simulink model "lab2_2"  (R2025b)
settings: Solver=FixedStepAuto  StartTime=0.0  StopTime=50.0  FixedStep=2^-7  RelTol=1e-3
settings Model: Creator=mizula  LastModifiedBy=mizula

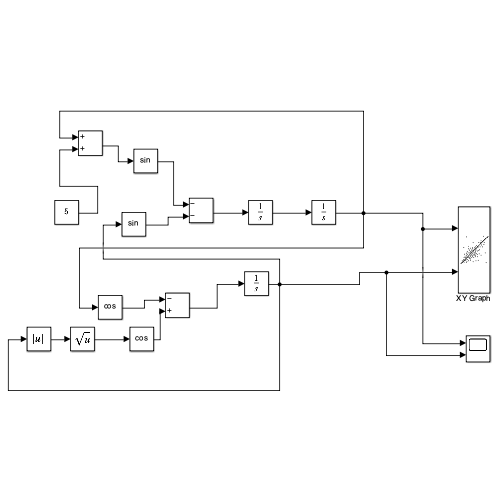
[thumbnail: Simulink's stored preview of the top-level diagram]
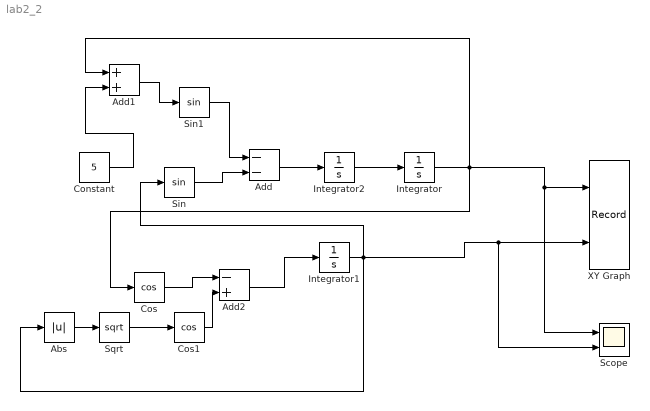
== system lab2_2 ==
  Abs : Abs  SaturateOnIntegerOverflow=off
  Add : Sum  Inputs=--
  Add1 : Sum
  Add2 : Sum  Inputs=-+
  Constant : Constant  Value=5
  Cos : Trigonometry  Operator=cos
  Cos1 : Trigonometry  Operator=cos
  Integrator : Integrator  InitialCondition=1
  Integrator1 : Integrator  InitialCondition=2
  Integrator2 : Integrator  InitialCondition=5
  Scope : Scope  NumInputPorts=2
      settings: ActiveDisplayYMinimum=-181.93688908773905  ActiveDisplayYMaximum=71.777306513933709
  Sin : Trigonometry
  Sin1 : Trigonometry
  Sqrt : Sqrt
  XY Graph : Record  NumPorts=2.0  FileSettingsInternal="{\"entries\":[{\"content\":{\"excelSettings\":{\"content\":{},\"type\":\"Streamout.ExcelSettings\"},\"parquetSettings\":{\"content\":{},\"type\":\"Streamout.ParquetSettings\"}},\"type\":\"Streamout.FileSettingStorage\",\"uuid\":\"\"}],\"packageUris\":[\"http:\\/\\/schema.mathworks.com\\/mf0\\/streamout_blocks\\/R2020a\"],\"version\":\"1.0\"}"  FrameSettings=[0, 0]  Layout=[1 1]  SignalsInternal="{\"entries\":[{\"content\":{\"signals\":[{\"content\":{\"blockPath\":[],\"dimensions\":[1],\"domain\":\"\",\"lineColor\":\"#a2142f\",\"plots\":[ 1 ],\"port\":1,\"sid\":[\"\"],\"signalID\":1,\"signalName\":\"Integrator\"},\"type\":\"RecordBlkView.Signal\",\"uuid\":\"\"},{\"content\":{\"blockPath\":[],\"dimensions\":[1],\"domain\":\"\",\"lineColor\":\"#139fff\",\"plots\":[ 1 ],\"port\":2,\"sid\":[\"\"],\"signalID\":2,\"signalName\":\"Integrator1\"},\"type\":\"RecordBlkView.Signal\",\"uuid\":\"\"}]},\"type\":\"RecordBlkView.InputSignals\",\"uuid\":\"\"}],\"packageUris\":[\"http:\\/\\/schema.mathworks.com\\/mf0\\/streamout_blocks\\/R2020a\"],\"version\":\"1.0\"}"  VisualizationBindings="{\"xyplotplugin\":{\"info\":[{\"series\":[{\"bindingParametersList\":[{\"parameter\":\"X-Axis\",\"signalID\":1,\"signalName\":\"Integrator\"},{\"parameter\":\"Y-Axis\",\"signalID\":2,\"signalName\":\"Integrator1\"}],\"seriesID\":0}],\"subplotID\":1}]}}"  CompatibilityTag=XY
  wires:
  Integrator1/1 -> Sin/1, Abs/1, Scope/2, XY Graph/2
  Sin/1 -> Add/2
  Integrator/1 -> Cos/1, Scope/1, XY Graph/1, Add1/1
  Add1/1 -> Sin1/1
  Sin1/1 -> Add/1
  Constant/1 -> Add1/2
  Add/1 -> Integrator2/1
  Cos/1 -> Add2/1
  Add2/1 -> Integrator1/1
  Cos1/1 -> Add2/2
  Sqrt/1 -> Cos1/1
  Integrator2/1 -> Integrator/1
  Abs/1 -> Sqrt/1
